simulink model "E_3"  (R2020a)
settings: Solver=VariableStepAuto  StartTime=0.0  StopTime=10  RelTol=1e-3
settings Model: Creator=Santiago  LastModifiedBy=Santiago

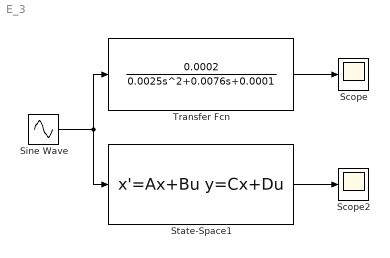
== system E_3 ==
  Scope : Scope
  Scope2 : Scope
  Sine Wave : Sin  Amplitude=120  Frequency=2*pi*60  SampleTime=0.00001
  State-Space1 : StateSpace  A=[-3 -2;-0.04 -0.04]  B=[0; 0.04]  C=[-1 0]  D=0  InitialCondition=0
  Transfer Fcn : TransferFcn  Numerator=[0.0002]  Denominator=[0.0025 0.0076 0.0001]
  wires:
  Sine Wave/1 -> Transfer Fcn/1, State-Space1/1
  Transfer Fcn/1 -> Scope/1
  State-Space1/1 -> Scope2/1
